simulink library "simlib_vpc_basic"  (R2022a)
settings: Solver=VariableStepAuto  StartTime=0.0  StopTime=10.0  RelTol=1e-3
undefined symbols (not defined in the file or in its folder): __PRM__SERIALIZED__DATA__, Ad, Camera, Pinhole, RBM, RRBM, VMO, VPC
libraries: $bdroot x10, simlib_vpc_coremath x5
(part 1 of 2)
settings Model: Creator=marco  LastModifiedBy=marco
settings SolverCC: AlgebraicLoopSolver=TrustRegion
settings DebuggingCC: UnconnectedInputMsg=warning  UnconnectedOutputMsg=warning  UnconnectedLineMsg=warning  SFMachineParentedDataDiag=warning
settings RTWCC: DLArmComputeVersion=19.05

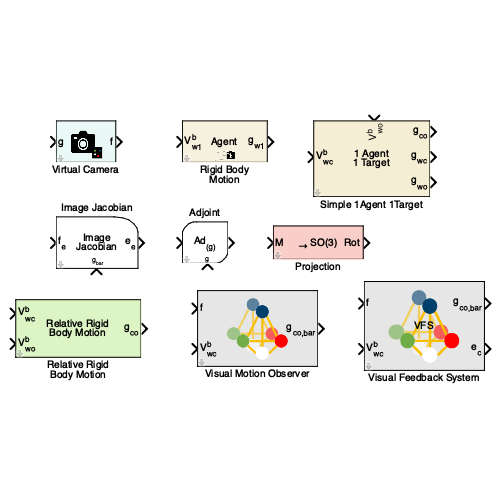
[thumbnail: Simulink's stored preview of the top-level diagram]
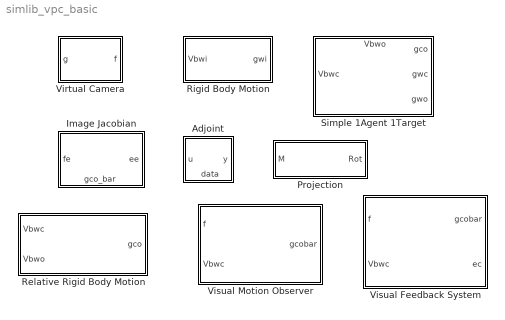
== system simlib_vpc_basic ==
  Adjoint : Subsystem  BlockKeywords=__PRM__SERIALIZED__DATA__:Ad  TreatAsAtomicUnit=on  mask(Adjoint Matrix [V1]){adjointtype=pose}
      mask prompts: adjointtype "Adjoint matrix is based on:"
      mask help:
      | Multiplies the Adjoint matrix with the input.
      | To calculate the Adjoint matrix, the position, orientation, or full pose must be given.
      settings: PortSchema="{\"entries\":[{\"content\":{\"sides\":[{\"content\":{\"connectorIds\":[\"In1\"]},\"type\":\"ConnectorPlacement.EquallySpacedRectSide\",\"uuid\":\"7e2da421-add1-40b5-9446-7b0ea0a4f10f\"},{\"content\":{\"connectorIds\":[\"Out1\"],\"side\":\"RIGHT\"},\"type\":\"ConnectorPlacement.EquallySpacedRectSide\",\"uuid\":\"b0158e1e-600a-48e8-a911-48a3898aac4e\"},{\"content\":{\"connectorIds\":[],\"side\":\"TOP\"},\"type\":\"ConnectorPlacement.EquallySpacedRectSide\",\"uuid\":\"4bc828d1-dee2-499b-9d21-a07f027570ae\"},{\"content\":{\"connectorIds\":[\"In2\"],\"side\":\"BOTTOM\"},\"type\":\"ConnectorPlacement.EquallySpacedRectSide\",\"uuid\":\"beed8369-7b41-42da-9d64-0cf6bc349210\"},{\"content\":{\"connectorIds\":[],\"side\":\"HIDDEN\"},\"type\":\"ConnectorPlacement.EquallySpacedRectSide\",\"uuid\":\"5ea700d9-1fcc-4187-8674-17f5733302d7\"}]},\"type\":\"ConnectorPlacement.EquallySpacedConnector\",\"uuid\":\"feef5c4e-af92-4970-8f4b-9fe20ba05ac5\"}],\"packageUris\":[\"http://schema.mathworks.com/mf0/Connector/R2020b\"],\"version\":\"1.0\"}"
      mask Help:
      | Refer to:
      | T. Hatanaka, N. Chopra, M. Fujita, and M. W. Spong, <i>Passivity-based Control and Estimation in Networked Robotics</i>, ser. Communications and Control Engineering. Springer, 2015.
      mask TypeOptions adjointtype: pose | position | orientation
      mask Display:
      | % Glitch in Matlab: If you define a line whose starting point and end point
      | % is equal, then the entire mask block is plotted in bold
      | plot([0,0],[0,0])
      | 
      | % Draw box
      | indent = 0.3;
      | ang=[0:0.2:pi/2, pi/2];
      | plot([0,1-indent],[0,0])
      | xp=indent*sin(ang)+1-indent;
      | yp=indent-indent*cos(ang);
      | plot(xp,yp);
      | plot([1,1,indent],[indent,1,1])
      | xp=indent-indent*sin(ang);
      | yp=1-indent+indent*cos(ang);
      | plot(xp,yp);
      | plot([0,0],[1-indent,0])
      | 
      | % Write label & ports
      | adjointtype = get_param(gcb, 'adjointtype');
      | porttype = '';
      | switch adjointtype
      |     case 'pose'
      |         disp('Ad_{(g)}','texmode','on')
      |         porttype = 'g';
      |     case 'position'
      |         disp('Ad_{(p)}','texmode','on')
      |         porttype = 'p';
      |     case 'orientation'
      |         disp('Ad_{(R)}','texmode','on')
      |         porttype = 'R';
      | end
      | switch get_param(gcb,'Orientation')
      |     case 'right'
      |         text(0.5,0.2,['\fontsize{7}' porttype],'texmode','on')
      |     case 'down'
      |         text(0.05,0.6,['\fontsize{7}' porttype],'texmode','on')
      |     case 'left'
      |         text(0.5,0.95,['\fontsize{7}' porttype],'texmode','on')
      |     case 'up'
      |         text(0.85,0.6,['\fontsize{7}' porttype],'texmode','on')
      | end
  Image Jacobian : Subsystem  TreatAsAtomicUnit=on  mask(Image Jacobian [V1]){po=[0, 10*sqrt(3), 0;15, -5*sqrt(3), 0;-15, -5*sqrt(3), 0;0, 0, 10*sqrt(6)]./100, lambda=0.0041}
      mask prompts: po "Feature point position coordinates (fixed in object frame Σo) [m]"; lambda "Focal length λ [m]"
      mask help:
      | Calculates the estimation error from the visual measurement error.
      | To that regard, the <i>Image Jacobian</i> is calculated, which itself depends on the VMO-estimate of the pose <i>gco</i>.
      |
      | Note: The focal length and feature point position coordinates in the object frame must be exactly known.
      settings: PortSchema="{\"entries\":[{\"content\":{\"sides\":[{\"content\":{\"connectorIds\":[\"In1\"]},\"type\":\"ConnectorPlacement.EquallySpacedRectSide\",\"uuid\":\"3d122c75-6063-48d0-bdc6-e48d95f4f0df\"},{\"content\":{\"connectorIds\":[\"Out1\"],\"side\":\"RIGHT\"},\"type\":\"ConnectorPlacement.EquallySpacedRectSide\",\"uuid\":\"6f2baba1-0bbd-4647-86ee-c97990dc6bd4\"},{\"content\":{\"connectorIds\":[],\"side\":\"TOP\"},\"type\":\"ConnectorPlacement.EquallySpacedRectSide\",\"uuid\":\"e6bc68d2-46ec-4597-a68e-7f59d26336ee\"},{\"content\":{\"connectorIds\":[\"In2\"],\"side\":\"BOTTOM\"},\"type\":\"ConnectorPlacement.EquallySpacedRectSide\",\"uuid\":\"b2d95be7-b34a-40bf-916a-28f2d4974c3e\"},{\"content\":{\"connectorIds\":[],\"side\":\"HIDDEN\"},\"type\":\"ConnectorPlacement.EquallySpacedRectSide\",\"uuid\":\"d66c6085-c61f-489e-b38a-36804ae2ee0b\"}]},\"type\":\"ConnectorPlacement.EquallySpacedConnector\",\"uuid\":\"9cb4cf54-89e1-4d8f-a4cb-7cce930f6af0\"}],\"packageUris\":[\"http://schema.mathworks.com/mf0/Connector/R2020b\"],\"version\":\"1.0\"}"
      mask Help:
      | Refer to:
      | T. Hatanaka, N. Chopra, M. Fujita, and M. W. Spong, <i>Passivity-based Control and Estimation in Networked Robotics</i>, ser. Communications and Control Engineering. Springer, 2015.
      mask Display:
      | % Glitch in Matlab: If you define a line whose starting point and end point
      | % is equal, then the entire mask block is plotted in bold
      | plot([0,0],[0,0])
      | 
      | % Draw box
      | indent = 0.3;
      | ang=[0:0.3:pi/2, pi/2];
      | xp=indent*cos(ang)+1-indent;
      | yp=indent*sin(ang)+1-indent;
      | plot([1,1,0,0,1-indent],[1-indent,0,0,1,1])
      | plot(xp,yp);
      | 
      | % Write label
      | % disp('J^{\spadesuit}(g_{co,bar})','texmode','on')
      | fprintf('Image\nJacobian','texmode','on')
      | 
      | % Label ports
      | port_label('input',1,'f_e','texmode','on')
      | % port_label('input',2,'g_{co,bar}','texmode','on')
      | text(0.45,0.2,'\fontsize{7}g_{bar}','texmode','on')
      | port_label('output',1,'e_e','texmode','on')
  Projection : Subsystem  TreatAsAtomicUnit=on  mask(Rotation Projection [V1]){projectiontype=averaging, inputtype=rotation matrix}
      mask prompts: projectiontype "Type of rotation projection:"; inputtype "Type of rotation input:"
      mask help:
      | This block projects an arbitrary matrix M [size 3x3] to the closest rotation matrix in SO3.
      |
      | Note:
      | Due to integration, a rotation matrix might only be "rotation"-like, as the determinant might change.
      | A real rotation matrix is orthogonal and has always determinant 1.
      | This block projects the input-matrix M to the closest rotation matrix R with such properties.
      mask Help:
      | Refer to:
      | T. Hatanaka, N. Chopra, M. Fujita, and M. W. Spong, <i>Passivity-based Control and Estimation in Networked Robotics</i>, ser. Communications and Control Engineering. Springer, 2015.
      mask TypeOptions projectiontype: averaging
      mask TypeOptions inputtype: rotation matrix | pose
      mask Display:
      | % Glitch in Matlab: If you define a line whose starting point and end point
      | % is equal, then the entire mask block is plotted in bold
      | plot([0,0],[0,0])
      | 
      | % Draw Box
      | plot([0,1,1,0,0],[0,0,1,1,0])
      | 
      | % Write label
      | disp('\rightarrow SO(3)','texmode','on')
      | 
      | % Label ports
      | inputtype = get_param(gcb, 'inputtype');
      | switch inputtype
      |     case 'rotation matrix'
      |         port_label('input',1,'M','texmode','on')
      |         port_label('output',1,'Rot','texmode','on')
      |     case 'pose'
      |         port_label('input',1,'g_M','texmode','on')
      |         port_label('output',1,'g','texmode','on')
      | end
  Relative Rigid Body Motion : Subsystem  BlockKeywords=__PRM__SERIALIZED__DATA__:RRBM  mask(Relative Rigid Body Motion Block [V1]){gco0=eye(4), projection=on, show_dgco=off}
      mask prompts: gco0 "Initial condition gco(0):"; projection "Use projection"; show_dgco "Show dgco"
      mask help: Relative rigid body motion of agent A as it can be observed from agent B.
      mask init:
      | block = find_system(gcb,'LookUnderMasks','on',...
      |     'FollowLinks','on','Name','Projection');
      | 
      | if projection && isempty(block) % Turn on projection
      |     % Delete lines
      |     delete_line(gcb,'Integrator/1','gco/1')
      |     delete_line(gcb,'Integrator/1','rrbm/3')
      |     
      |     % Add block
      |     add_block([bdroot(gcb),'/Projection'],[gcb,'/Projection'],'inputtype','pose');
      |     
      |     % Connect lines
      |     add_line(gcb,'Integrator/1','Projection/1','autorouting','smart')
      |     add_line(gcb,'Projection/1','gco/1','autorouting','smart')
      |     add_line(gcb,'Projection/1','rrbm/3','autorouting','smart')
      | elseif ~projection && ~isempty(block) % Turn off projection
      |     % Delete lines
      |     delete_line(gcb,'Integrator/1','Projection/1')
      |     delete_line(gcb,'Projection/1','gco/1')
      |     delete_line(gcb,'Projection/1','rrbm/3')
      | 
      |     % Delete block
      |     delete_block(block);
      | 
      |     % Connect blocks
      |     add_line(gcb,'Integrator/1','gco/1','autorouting','smart')
      |     add_line(gcb,'Integrator/1','rrbm/3','autorouting','smart')
      | end
      | 
      | % Show dgco output
      | if show_dgco
      |     % Add block & lines
      |     try; add_block('built-in/Outport',[gcb,'/dgco'],'Port','2','Position',[510 193 540 207]); end;
      |     try; add_line(gcb,'rrbm/1','dgco/1','autorouting','smart'); end;
      | else
      |     % Delete block & lines
      |     dgcoblock = find_system(gcb,'SearchDepth','1','LookUnderMasks','on',...
      |         'FollowLinks','on','Name','dgco');
      |     try; delete_line(gcb,'rrbm/1','dgco/1'); end;
      |     try; delete_block(dgcoblock); end;
      | end
      settings: MinAlgLoopOccurrences=on
      mask Help:
      | Refer to:
      | T. Hatanaka, N. Chopra, M. Fujita, and M. W. Spong, <i>Passivity-based Control and Estimation in Networked Robotics</i>, ser. Communications and Control Engineering. Springer, 2015.
      mask TypeOptions gco0: Integrator/InitialCondition
      mask DialogControl show_dgco Tooltip: If on, the internal state derivative of gco will be shown as an output
      mask Display:
      | % Glitch in Matlab: If you define a line whose starting point and end point
      | % is equal, then the entire mask block is plotted in bold
      | plot([0,0],[0,0])
      | 
      | % Draw Box
      | plot([0,1,1,0,0],[0,0,1,1,0])
      | 
      | % Write label
      | fprintf('Relative Rigid\nBody Motion','texmode','on')
      | 
      | % Label ports
      | port_label('input',1,'V^{b}_{wc}','texmode','on')
      | port_label('input',2,'V^{b}_{wo}','texmode','on')
      | port_label('output',1,'g_{co}','texmode','on')
      | if strcmp(get_param(gcb,'show_dgco'),'on')
      |     port_label('output',2,'dg_{co}','texmode','on')
      | end
  Rigid Body Motion : Subsystem  BlockKeywords=__PRM__SERIALIZED__DATA__:RBM  mask(Rigid Body Motion Block [V1]){rbmtype=agent, agentnumber=1, projection=on, show_dg=off, g0=eye(4)}
      mask prompts: rbmtype "Type:"; agentnumber "#"; projection "Use projection"; show_dg "Show derivative dg"; g0 "Initial condition g(0):"
      mask help:
      | Implements a simple (single-integrator-type) rigid body motion model.
      | The RBM type in the parameter pane is just for a better visualization purpose and does not have any effect on the dynamics, but the block mask appearance.
      mask init:
      | block = find_system(gcb,'LookUnderMasks','on',...
      |     'FollowLinks','on','Name','Projection');
      | 
      | if projection && isempty(block) % Turn on projection
      |     % Delete lines
      |     delete_line(gcb,'Integrator/1','gwi/1')
      |     delete_line(gcb,'Integrator/1','rbm/2')
      |     
      |     % Add block
      |     add_block([bdroot(gcb),'/Projection'],[gcb,'/Projection'],'inputtype','pose');
      |     
      |     % Connect lines
      |     add_line(gcb,'Integrator/1','Projection/1','autorouting','smart')
      |     add_line(gcb,'Projection/1','gwi/1','autorouting','smart')
      |     add_line(gcb,'Projection/1','rbm/2','autorouting','smart')
      | elseif ~projection && ~isempty(block) % Turn off projection
      |     % Delete lines
      |     delete_line(gcb,'Integrator/1','Projection/1')
      |     delete_line(gcb,'Projection/1','gwi/1')
      |     delete_line(gcb,'Projection/1','rbm/2')
      | 
      |     % Delete block
      |     delete_block(block);
      | 
      |     % Connect blocks
      |     add_line(gcb,'Integrator/1','gwi/1','autorouting','smart')
      |     add_line(gcb,'Integrator/1','rbm/2','autorouting','smart')
      | end
      | 
      | % Show derivative output dg
      | if show_dg
      |     % Add block & lines
      |     try; add_block('built-in/Outport',[gcb,'/dgwi'],'Port','2','Position',[515 203 545 217]); end;
      |     try; add_line(gcb,'rbm/1','dgwi/1','autorouting','smart'); end;
      | else
      |     % Delete block & lines
      |     dgwiblock = find_system(gcb,'SearchDepth','1','LookUnderMasks','on',...
      |         'FollowLinks','on','Name','dgwi');
      |     try; delete_line(gcb,'rbm/1','dgwi/1'); end;
      |     try; delete_block(dgwiblock); end;
      | end
      settings: MinAlgLoopOccurrences=on
      mask Help:
      | Refer to:
      | T. Hatanaka, N. Chopra, M. Fujita, and M. W. Spong, <i>Passivity-based Control and Estimation in Networked Robotics</i>, ser. Communications and Control Engineering. Springer, 2015.
      mask TypeOptions rbmtype: agent | target
      mask Callback rbmtype:
      | rbmtype = get_param(gcb,'rbmtype');
      | 
      | switch rbmtype
      |     case 'agent'
      |         % Turn on number field
      |         set_param(gcb,'MaskVisibilities',{'on';'on';'on';'on';'on'});
      |     case 'target'
      |         % Turn off number field
      |         set_param(gcb,'MaskVisibilities',{'on';'off';'on';'on';'on'});
      |         % Set number in the invisible field to 0
      |         % set_param(gcb,'agentnumber','0');
      | end
      mask Display:
      | % Glitch in Matlab: If you define a line whose starting point and end point
      | % is equal, then the entire mask block is plotted in bold
      | plot([0,0],[0,0])
      | 
      | % Draw Box
      | plot([0,1,1,0,0],[0,0,1,1,0])
      | 
      | % Write label
      | rbmtype = get_param(gcb, 'rbmtype');
      | switch rbmtype
      |     case 'agent'
      |         agentnumber = get_param(gcb, 'agentnumber');
      |         disp('Agent','texmode','on')
      | 
      |         % Image
      |         p=get_param(gcb,'Position');
      |         size = min(p(3:4)-p(1:2));
      |         blkscale = abs((p(3)-p(1)) / (p(4)-p(2)));
      |         if abs((p(3)-p(1))) > abs((p(4)-p(2))) % block is horizontal
      |             scale = .5*[1/blkscale .6];
      |         else % block is vertical
      |             scale = .5*[1 .6*blkscale];
      |         end
      |         pos = [1-scale(1) 0.1]/2;
      |         image('ico_agent.png',[pos scale],'off')
      |     case 'target'
      |         agentnumber = 0;
      |         disp('Target','texmode','on')
      | 
      |         % Image
      |         p=get_param(gcb,'Position');
      |         size = min(p(3:4)-p(1:2));
      |         blkscale = abs((p(3)-p(1)) / (p(4)-p(2)));
      |         if abs((p(3)-p(1))) > abs((p(4)-p(2))) % block is horizontal
      |             scale = .5*[1/blkscale .6];
      |         else % block is vertical
      |             scale = .5*[1 .6*blkscale];
      |         end
      |         pos = [1-scale(1) 0.1]/2;
      |         image('ico_target.png',[pos scale],'off')
      | end
      | 
      | % Label ports
      | port_label('input',1,['V^{b}_{w' num2str(agentnumber) '}'],'texmode','on')
      | port_label('output',1,['g_{w' num2str(agentnumber) '}'],'texmode','on')
      | if strcmp(get_param(gcb, 'show_dg'),'on')
      |     port_label('output',2,['dg_{w' num2str(agentnumber) '}'],'texmode','on')
      | end
  Simple 1Agent 1Target : Subsystem  mask(Simple 1Agent 1 Target block [V1]){gwc0=eye(4), projectionAgent=on, gwo0=eye(4), projectionTarget=on, showgwc=on, showdgwc=off, showgwo=on, showdgwo=off}
      mask prompts: gwc0 "Initial condition gwc(0):"; projectionAgent "Use projection"; gwo0 "Initial condition gwo(0):"; projectionTarget "Use projection"; showgwc "Output gwc"; showdgwc "Output dgwc"; showgwo "Output gwo"; showdgwo "Output dgwo"
      mask help: Implements a simple relative rigid body motion block with one target and one agent.
      mask init:
      | % Blocks
      | gwcblock = find_system(gcb,'LookUnderMasks','on',...
      |     'FollowLinks','on','Name','gwc');
      | dgwcblock = find_system(gcb,'LookUnderMasks','on',...
      |     'FollowLinks','on','Name','dgwc');
      | gwoblock = find_system(gcb,'LookUnderMasks','on',...
      |     'FollowLinks','on','Name','gwo');
      | dgwoblock = find_system(gcb,'LookUnderMasks','on',...
      |     'FollowLinks','on','Name','dgwo');
      | 
      | portnum = 2;
      | 
      | if showgwc % Output gwc
      |     % Add block
      |     try; add_block('built-in/Outport',[gcb,'/gwc'],'Position',[380 128 410 142],'Port',num2str(portnum)); end;
      |     portnum = portnum + 1;
      |     % Connect lines
      |     try; add_line(gcb,'Agent/1','gwc/1','autorouting','smart'); end;
      | else % Hide gwc
      |     % Delete lines
      |     try; delete_line(gcb,'Agent/1','gwc/1'); end;
      |     % Delete block
      |     try; delete_block(gwcblock); end;
      | end
      | 
      | if showdgwc % Output dgwc
      |     % Pass argument to agent block
      |     set_param([gcb,'/Agent'],'show_dg','on')
      |     % Add block
      |     try; add_block('built-in/Outport',[gcb,'/dgwc'],'Position',[200 148 230 162],'Port',num2str(portnum)); end;
      |     portnum = portnum + 1;
      |     % Connect lines
      |     try; add_line(gcb,'Agent/2','dgwc/1','autorouting','smart'); end;
      | else % Hide dgwc
      |     % Delete lines
      |     try; delete_line(gcb,'Agent/2','dgwc/1'); end;
      |     % Delete block
      |     try; delete_block(dgwcblock); end;
      |     % Pass argument to agent block
      |     set_param([gcb,'/Agent'],'show_dg','off')
      | end
      | 
      | if showgwo % Output gwc
      |     % Add block
      |     try; add_block('built-in/Outport',[gcb,'/gwo'],'Position',[380 48 410 62],'Port',num2str(portnum)); end;
      |     portnum = portnum + 1;
      |     % Connect lines
      |     try; add_line(gcb,'Target/1','gwo/1','autorouting','smart'); end;
      | else % Hide gwc
      |     % Delete lines
      |     try; delete_line(gcb,'Target/1','gwo/1'); end;
      |     % Delete block
      |     try; delete_block(gwoblock); end;
      | end
      | 
      | if showdgwo % Output dgwo
      |     % Pass argument to target block
      |     set_param([gcb,'/Target'],'show_dg','on')
      |     % Add block
      |     try; add_block('built-in/Outport',[gcb,'/dgwo'],'Position',[200 63 230 77],'Port',num2str(portnum)); end;
      |     portnum = portnum + 1;
      |     % Connect lines
      |     try; add_line(gcb,'Target/2','dgwo/1','autorouting','smart'); end;
      | else % Hide dgwo
      |     % Delete lines
      |     try; delete_line(gcb,'Target/2','dgwo/1'); end;
      |     % Delete block
      |     try; delete_block(dgwoblock); end;
      |     % Pass argument to agent block
      |     set_param([gcb,'/Target'],'show_dg','off')
      | end
      settings: PortSchema="{\"entries\":[{\"content\":{\"sides\":[{\"content\":{\"connectorIds\":[\"In1\"]},\"type\":\"ConnectorPlacement.EquallySpacedRectSide\",\"uuid\":\"51848c78-49bf-4d69-8138-12848c04a52b\"},{\"content\":{\"connectorIds\":[\"Out1\",\"Out2\",\"Out3\"],\"side\":\"RIGHT\"},\"type\":\"ConnectorPlacement.EquallySpacedRectSide\",\"uuid\":\"a2771237-d1b3-407b-8d53-6a34779e1c0e\"},{\"content\":{\"connectorIds\":[\"In2\"],\"side\":\"TOP\"},\"type\":\"ConnectorPlacement.EquallySpacedRectSide\",\"uuid\":\"c6712b15-7cf3-4a58-80e7-6bd7851abb53\"},{\"content\":{\"connectorIds\":[],\"side\":\"HIDDEN\"},\"type\":\"ConnectorPlacement.EquallySpacedRectSide\",\"uuid\":\"8616ed9a-8306-41f0-bffd-55839930ff42\"}]},\"type\":\"ConnectorPlacement.EquallySpacedConnector\",\"uuid\":\"4f48229c-43f3-4c05-9119-4c52932f0077\"}],\"packageUris\":[\"http://schema.mathworks.com/mf0/Connector/R2020b\"],\"version\":\"1.0\"}"
      mask Help:
      | Refer to:
      | T. Hatanaka, N. Chopra, M. Fujita, and M. W. Spong, <i>Passivity-based Control and Estimation in Networked Robotics</i>, ser. Communications and Control Engineering. Springer, 2015.
      mask TypeOptions gwc0: Agent/g0
      mask TypeOptions projectionAgent: Agent/projection
      mask TypeOptions gwo0: Target/g0
      mask TypeOptions projectionTarget: Target/projection
      mask DialogControl AgentParameters Prompt: Agent Parameters
      mask DialogControl TargetParameters Prompt: Target Parameters
      mask DialogControl OutputPorts Prompt: Auxiliary outputs
      mask Display:
      | % Glitch in Matlab: If you define a line whose starting point and end point
      | % is equal, then the entire mask block is plotted in bold
      | plot([0,0],[0,0])
      | 
      | % Draw Box
      | plot([0,1,1,0,0],[0,0,1,1,0])
      | 
      | % Write label
      | fprintf('1 Agent\n1 Target','texmode','on')
      | 
      | % Label ports
      | port_label('input',1,'V^{b}_{wc}','texmode','on')
      | port_label('input',2,'V^{b}_{wo}','texmode','on')
      | port_label('output',1,'g_{co}','texmode','on')
      | 
      | % Label dynamic output ports
      | portnumber = 2;
      | if strcmp(get_param(gcb, 'showgwc'),'on')
      |     port_label('output',portnumber,'g_{wc}','texmode','on')
      |     portnumber = portnumber + 1;
      | end
      | if strcmp(get_param(gcb, 'showdgwc'),'on')
      |     port_label('output',portnumber,'dg_{wc}','texmode','on')
      |     portnumber = portnumber + 1;
      | end
      | if strcmp(get_param(gcb, 'showgwo'),'on')
      |     port_label('output',portnumber,'g_{wo}','texmode','on')
      |     portnumber = portnumber + 1;
      | end
      | if strcmp(get_param(gcb, 'showdgwo'),'on')
      |     port_label('output',portnumber,'dg_{wo}','texmode','on')
      |     portnumber = portnumber + 1;
      | end
  Virtual Camera : Subsystem  BlockKeywords=__PRM__SERIALIZED__DATA__:Camera  TreatAsAtomicUnit=on  mask(Virtual Camera model [V1]){camtype=Pinhole, po=[0, 10*sqrt(3), 0;15, -5*sqrt(3), 0;-15, -5*sqrt(3), 0;0, 0, 10*sqrt(6)]./100, lambda=0.0041}
      mask prompts: camtype "Camera type"; po "Feature point position coordinates (fixed in object frame Σo) [m]"; lambda "Focal length λ [m]"
      mask help:
      | A simple virtual camera model.
      | Outputs feature points in image-coordinates.
      |
      | Note: So far, only a virtual "Pinhole" camera model is implemented.
      mask Help:
      | Refer to:
      | T. Hatanaka, N. Chopra, M. Fujita, and M. W. Spong, <i>Passivity-based Control and Estimation in Networked Robotics</i>, ser. Communications and Control Engineering. Springer, 2015.
      mask TypeOptions camtype: Pinhole
      mask Display:
      | % Glitch in Matlab: If you define a line whose starting point and end point
      | % is equal, then the entire mask block is plotted in bold
      | plot([0,0],[0,0])
      | 
      | % Draw Box
      | plot([0,1,1,0,0],[0,0,1,1,0])
      | 
      | % Write label
      | % disp('Camera','texmode','on')
      | p=get_param(gcb,'Position');
      | size = min(p(3:4)-p(1:2));
      | blkscale = abs((p(3)-p(1)) / (p(4)-p(2)));
      | if abs((p(3)-p(1))) > abs((p(4)-p(2))) % block is horizontal
      |     scale = .8*[1/blkscale 1];
      | else % block is vertical
      |     scale = .8*[1 blkscale];
      | end
      | pos = [1-scale(1) 1-scale(2)]./2;
      | image('ico_vis.png',[pos scale],'off')
      | 
      | % Label ports
      | port_label('input',1,'g','texmode','on')
      | port_label('output',1,'f','texmode','on')
  Visual Feedback System : Subsystem  BlockKeywords=__PRM__SERIALIZED__DATA__:VPC  mask(Visual Pursuit Control [V1]){gd_source=internal, gd_value=[eye(4,3),ones(4,1)], gcobar0=[eye(4,3), ones(4,1)], Ke_source=internal, Ke=5*eye(6), projection=on, camtype=Pinhole, fo=[0, 10*sqrt(3), 0;15, -5*sqrt(3), 0;-15, -5*sqrt(3), 0;0, 0, 10*sqrt(6)]./100, lambda=0.0041, show_Vbwo=off, show_ec=on, show_gce=off, show_ee=off, show_gee=off, show_e=off, show_nu=off, show_dgcobar=off, show_ue_aux=off}
      mask prompts: gd_source "Desired pose source:"; gd_value "Desired pose"; gcobar0 "Initial estimate gco_bar(0):"; Ke_source "Observer gain source:"; Ke "Observer gain Ke"; projection "Use projection"; camtype "Camera type"; fo "Feature point position coordinates (fixed in object frame Σo) [m]"; lambda "Camera focal length λ [m]"; show_Vbwo "estimated target velocity Vbwo"; show_ec "control error ec"; show_gce "control error gce"; show_ee "estimation error ee"; show_gee "estimation error gee"; show_e "total error e"; show_nu "nu"; show_dgcobar "estimation derivative"; show_ue_aux "feed-forward ue"
      mask help:
      | Visual Feedback System block.
      | Implements the visual pursuit control scheme. Has the visual motion observer block included.
      | Check parameters carefully.
      mask init:
      | % Switch gd: external <-> internal
      | port_number = 3;
      | switch gd_source
      |     case 1 % Make internal
      |         % Delete block & lines
      |         gd = find_system(gcb,'SearchDepth','1','LookUnderMasks','on',...
      |             'FollowLinks','on','Name','gd_inport');
      |         try; delete_line(gcb,'gd_inport/1','Relative Pose/1'); end;
      |         try; delete_block(gd); end;
      | 
      |         % Add block & lines
      |         try; add_block('built-in/Constant',[gcb,'/Desired Pose'],'Value','gd_value','Position',[190 -291 285 -269]); end;
      |         try; add_line(gcb,'Desired Pose/1','Relative Pose/1','autorouting','smart'); end;
      |     case 2 % Make external
      |         % Delete block & lines
      |         gd = find_system(gcb,'SearchDepth','1','LookUnderMasks','on',...
      |             'FollowLinks','on','Name','Desired Pose');
      |         try; delete_line(gcb,'Desired Pose/1','Relative Pose/1'); end;
      |         try; delete_block(gd); end;
      | 
      |         % Add block & lines
      |         try; add_block('built-in/Inport',[gcb,'/gd_inport'],'Port',num2str(port_number),'Position',[220 -287 250 -273]); end;
      |         port_number = port_number + 1;
      |         try; add_line(gcb,'gd_inport/1','Relative Pose/1','autorouting','smart'); end;
      | end
      | 
      | % Switch Ke: external <-> internal
      | switch Ke_source
      |     case 1 % Make internal
      |         % Delete block & lines
      |         Ke_inport = find_system(gcb,'SearchDepth','1','LookUnderMasks','on',...
      |             'FollowLinks','on','Name','Ke_inport');
      |         Ke_mult = find_system(gcb,'SearchDepth','1','LookUnderMasks','on',...
      |             'FollowLinks','on','Name','Ke_mult');
      |         try; delete_line(gcb,'Demux/2','Ke_mult/2'); end;
      |         try; delete_line(gcb,'Ke_inport/1','Ke_mult/1'); end;
      |         try; delete_line(gcb,'Ke_mult/1','Gain/1'); end;
      |         try; delete_block(Ke_mult); end;
      |         try; delete_block(Ke_inport); end;
      | 
      |         % Add block & lines
      |         try; add_block('built-in/Gain',[gcb,'/Ke_gain'],'Gain','Ke','Multiplication','Matrix(K*u) (u vector)','Position',[175 -48 250 28],'Orientation','left'); end;
      |         try; add_line(gcb,'Demux/2','Ke_gain/1','autorouting','smart'); end;
      |         try; add_line(gcb,'Ke_gain/1','Gain/1','autorouting','smart'); end;
      |     case 2 % Make external
      |         % Delete block & lines
      |         Ke_gain = find_system(gcb,'SearchDepth','1','LookUnderMasks','on',...
      |             'FollowLinks','on','Name','Ke_gain');
      |         try; delete_line(gcb,'Demux/2','Ke_gain/1'); end;
      |         try; delete_line(gcb,'Ke_gain/1','Gain/1'); end;
      |         try; delete_block(Ke_gain); end;
      | 
      |         % Add block & lines
      |         try; add_block('built-in/Inport',[gcb,'/Ke_inport'],'Position',[255 -42 285 -28],'Port',num2str(port_number),'Orientation','left'); end;
      |         port_number = port_number + 1;
      |         try; add_block('built-in/Product',[gcb,'/Ke_mult'],'Multiplication','Matrix(*)','Position',[160 -50 210 5],'Orientation','left'); end;
      |         try; add_line(gcb,'Ke_inport/1','Ke_mult/1','autorouting','smart'); end;
      |         try; add_line(gcb,'Demux/2','Ke_mult/2','autorouting','smart'); end;
      |         try; add_line(gcb,'Ke_mult/1','Gain/1','autorouting','smart'); end;
      | end
      | 
      | % Show / Hide: ue_aux
      | if show_ue_aux % Show input
      |     % Delete block & lines
      |     try; delete_line(gcb,'Gain/1','Gain_ue/1'); end;
      | 
      |     % Add block & lines
      |     try; add_block('built-in/Inport',[gcb,'/ue_aux'],'Port',num2str(port_number),'Position',[-150 -132 -120 -118]); end;
      |     try; add_block('built-in/sum',[gcb,'/sum_ue'],'IconShape','round','Position',[-90 -135 -70 -115],'Inputs','|++'); end;
      |     try; add_line(gcb,'ue_aux/1','sum_ue/1','autorouting','smart'); end;
      |     try; add_line(gcb,'Gain/1','sum_ue/2','autorouting','smart'); end;
      |     try; add_line(gcb,'sum_ue/1','Gain_ue/1','autorouting','smart'); end;
      | else % Hide input
      |     % Delete block & lines
      |     ue = find_system(gcb,'SearchDepth','1','LookUnderMasks','on',...
      |         'FollowLinks','on','Name','ue_aux');
      |     sumblock = find_system(gcb,'SearchDepth','1','LookUnderMasks','on',...
      |         'FollowLinks','on','Name','sum_ue');
      |     try; delete_line(gcb,'ue_aux/1','sum_ue/1'); end;
      |     try; delete_line(gcb,'Gain/1','sum_ue/2'); end;
      |     try; delete_line(gcb,'sum_ue/1','Gain_ue/1'); end;
      |     try; delete_block(ue); end;
      |     try; delete_block(sumblock); end;
      | 
      |     % Add block & lines
      |     try; add_line(gcb,'Gain/1','Gain_ue/1','autorouting','smart'); end;
      | end
      | 
      | 
      | %%%%%%%%%%%%%%%%%%
      | %% Outputs
      | %%%%%%%%%%%%%%%%%%
      | port_number = 2;
      | 
      | % Show / Hide: Vbwo
      | if show_Vbwo % Show output
      |     try add_block('built-in/Outport',[gcb,'/Vbwo,bar'],'Port',num2str(port_number),'Position',[35 -77 65 -63]); catch; end
      |     try add_line(gcb,'Gain_ue/1','Vbwo,bar/1','autorouting','smart'); catch; end
      |     port_number = port_number+1;
      | else % Hide output
      |     block = find_system(gcb,'SearchDepth','1','LookUnderMasks','on',...
      |         'FollowLinks','on','Name','Vbwo,bar');
      |     try delete_line(gcb,'Gain_ue/1','Vbwo,bar/1'); catch; end
      |     try delete_block(block); catch; end
      | end
      | 
      | % Show / Hide: ec
      | if show_ec % Show output
      |     % Add block & lines
      |     try add_block('built-in/Outport',[gcb,'/ec'],'Port',num2str(port_number),'Position',[515 -262 545 -248]); catch; end
      |     try add_line(gcb,'vec/1','ec/1','autorouting','smart'); catch; end
      |     port_number = port_number + 1;
      | else % Hide output
      |     % Delete block & lines
      |     block = find_system(gcb,'SearchDepth','1','LookUnderMasks','on',...
      |         'FollowLinks','on','Name','ec');
      |     try delete_line(gcb,'vec/1','ec/1'); catch; end
      |     try delete_block(block); catch; end
      | end
      | 
      | % Show / Hide: ee
      | if show_ee % Show output
      |     try; add_block('built-in/Outport',[gcb,'/ee'],'Port',num2str(port_number),'Position',[515 -122 545 -108]); end;
      |     port_number = port_number + 1;
      |     try; add_line(gcb,'Image Jacobian/1','ee/1','autorouting','smart'); end;
      | else % Hide output
      |     ee = find_system(gcb,'SearchDepth','1','LookUnderMasks','on',...
      |         'FollowLinks','on','Name','ee');
      |     try; delete_line(gcb,'Image Jacobian/1','ee/1'); end;
      |     try; delete_block(ee); end;
      | end
      | 
      | % Show / Hide: gce
      | if show_gce % Show output
      |     try; add_block('built-in/Outport',[gcb,'/gce'],'Port',num2str(port_number),'Position',[515 -332 545 -318]); end;
      |     port_number = port_number + 1;
      |     try; add_line(gcb,'Relative Pose/1','gce/1','autorouting','smart'); end;
      | else % Hide output
      |     gce = find_system(gcb,'SearchDepth','1','LookUnderMasks','on',...
      |         'FollowLinks','on','Name','gce');
      |     try; delete_line(gcb,'Relative Pose/1','gce/1'); end;
      |     try; delete_block(gce); end;
      | end
      | 
      | % Show / Hide: gee
      | if show_gee % Show output
      |     block = find_system(gcb,'SearchDepth','1','LookUnderMasks','on',...
      |         'FollowLinks','on','Name','Terminator_gee');
      |     try delete_line(gcb,'unvec/1','Terminator_gee/1'); catch; end
      |     try delete_block(block); catch; end
      |     try add_block('built-in/Outport',[gcb,'/gee'],'Port',num2str(port_number),'Position',[645 -62 675 -48]); catch; end
      |     try add_line(gcb,'unvec/1','gee/1','autorouting','smart'); catch; end
      |     port_number = port_number+1;
      | else % Hide output
      |     block = find_system(gcb,'SearchDepth','1','LookUnderMasks','on',...
      |         'FollowLinks','on','Name','gee');
      |     try delete_line(gcb,'unvec/1','gee/1'); catch; end
      |     try delete_block(block); catch; end
      |     try add_block('built-in/Terminator',[gcb,'/Terminator_gee'],'Position',[645 -62 675 -48]); catch; end
      |     try add_line(gcb,'unvec/1','Terminator_gee/1','autorouting','smart'); catch; end
      | end
      | 
      | % Show / Hide: e
      | if show_e % Show output
      |     try; add_block('built-in/Outport',[gcb,'/e'],'Port',num2str(port_number),'Position',[660 -177 690 -163]); end;
      |     port_number = port_number + 1;
      |     try; add_line(gcb,'Vector Concatenate/1','e/1','autorouting','smart'); end;
      | else % Hide output
      |     e = find_system(gcb,'SearchDepth','1','LookUnderMasks','on',...
      |         'FollowLinks','on','Name','e');
      |     try; delete_line(gcb,'Vector Concatenate/1','e/1'); end;
      |     try; delete_block(e); end;
      | end
      | 
      | % Show / Hide: nu
      | if show_nu % Show output
      |     try; add_block('built-in/Outport',[gcb,'/nu'],'Port',num2str(port_number),'Position',[860 -242 890 -228]); end;
      |     port_number = port_number + 1;
      |     try; add_line(gcb,'Matrix Multiply/1','nu/1','autorouting','smart'); end;
      | else % Hide output
      |     nu = find_system(gcb,'SearchDepth','1','LookUnderMasks','on',...
      |         'FollowLinks','on','Name','nu');
      |     try; delete_line(gcb,'Matrix Multiply/1','nu/1'); end;
      |     try; delete_block(nu); end;
      | end
      | 
      | % Show / Hide: dgcobar
      | if show_dgcobar % Show output
      |     % Pass argument to rrbm block
      |     set_param([gcb,'/RRBM'],'show_dgco','on')
      |     % Add block & lines
      |     try; add_block('built-in/Outport',[gcb,'/dgcobar'],'Port',num2str(port_number),'Position',[225 -77 255 -63]); end;
      |     try; add_line(gcb,'RRBM/2','dgcobar/1','autorouting','smart'); end;
      | else
      |     % Delete block & lines
      |     dgcobarblock = find_system(gcb,'SearchDepth','1','LookUnderMasks','on',...
      |         'FollowLinks','on','Name','dgcobar');
      |     try; delete_line(gcb,'RRBM/2','dgcobar/1'); end;
      |     try; delete_block(dgcobarblock); end;
      |     % Pass argument to rrbm block
      |     set_param([gcb,'/RRBM'],'show_dgco','off')
      | end
      settings: MinAlgLoopOccurrences=on
      mask Help:
      | Refer to:
      | T. Hatanaka, N. Chopra, M. Fujita, and M. W. Spong, <i>Passivity-based Control and Estimation in Networked Robotics</i>, ser. Communications and Control Engineering. Springer, 2015.
      mask TypeOptions gd_source: internal | external
      mask Callback gd_source:
      | gd_source = get_param(gcb,'gd_source');
      | 
      | idx = find(strcmp(get_param(gcb,'MaskNames'),'gd_value'));
      | maskvis = get_param(gcb,'MaskVisibilities');
      | switch gd_source
      |     case 'internal' % Show gd field
      |         maskvis{idx} = 'on';
      |     case 'external' % Hide gd field
      |         maskvis{idx} = 'off';
      | end
      | set_param(gcb,'MaskVisibilities',maskvis);
      mask TypeOptions gcobar0: RRBM/gco0
      mask TypeOptions Ke_source: internal | external
      mask Callback Ke_source:
      | Ke_source = get_param(gcb,'Ke_source');
      | 
      | idx = find(strcmp(get_param(gcb,'MaskNames'),'Ke'));
      | maskvis = get_param(gcb,'MaskVisibilities');
      | switch Ke_source
      |     case 'internal' % Show Ke field
      |         maskvis{idx} = 'on';
      |     case 'external' % Hide Ke field
      |         maskvis{idx} = 'off';
      | end
      | set_param(gcb,'MaskVisibilities',maskvis);
      mask TypeOptions projection: RRBM/projection
      mask TypeOptions camtype: Virtual Camera/camtype
      mask TypeOptions fo: Virtual Camera/po
      mask TypeOptions lambda: Virtual Camera/lambda
      mask DialogControl VPCParameters Prompt: VPC Parameters
      mask DialogControl VMOParameters Prompt: VMO Parameters
      mask DialogControl CameraParameters Prompt: Camera Parameters
      mask DialogControl IOGroupVar Prompt: Show I/O
      mask DialogControl io_text Prompt: Tick the following checkboxes to show the corresponding inputs and outputs on the block.
      mask DialogControl Container7 Prompt: Outputs
      mask DialogControl show_gce Tooltip: If on, the pose control error gce will be shown at the output.
      mask DialogControl show_dgcobar Tooltip: If on, the estimation derivative dgcobar will be shown on the output.
      mask DialogControl Container8 Prompt: Inputs
      mask Display:
      | % Glitch in Matlab: If you define a line whose starting point and end point
      | % is equal, then the entire mask block is plotted in bold
      | plot([0,0],[0,0])
      | 
      | % Draw Box
      | plot([0,1,1,0,0],[0,0,1,1,0])
      | 
      | % Write label
      | p=get_param(gcb,'Position');
      | size = min(p(3:4)-p(1:2));
      | blkscale = abs((p(3)-p(1)) / (p(4)-p(2)));
      | if abs((p(3)-p(1))) > abs((p(4)-p(2))) % block is horizontal
      |     scale = .8*[1/blkscale 1];
      | else % block is vertical
      |     scale = .8*[1 blkscale];
      | end
      | pos = [1-scale(1) 1-scale(2)]./2;
      | image('ico_vmo.png',[pos scale],'off')
      | disp('VFS','texmode','on')
      | 
      | % Label input ports
      | port_label('input',1,'f','texmode','on')
      | port_label('input',2,'V^{b}_{wc}','texmode','on')
      | inport = 3;
      | if strcmp(get_param(gcb, 'gd_source'),'external')
      |     port_label('input',inport,'g_d','texmode','on')
      |     inport = inport + 1;
      | end
      | if strcmp(get_param(gcb, 'Ke_source'),'external')
      |     port_label('input',outport,'K_e','texmode','on')
      |     inport = inport + 1;
      | end
      | if strcmp(get_param(gcb, 'show_ue_aux'),'on')
      |     port_label('input',inport,'u_{e,aux}','texmode','on')
      |     inport = inport + 1;
      | end
      | 
      | % Label output ports
      | port_label('output',1,'g_{co,bar}','texmode','on')
      | outport = 2;
      | if strcmp(get_param(gcb, 'show_Vbwo'),'on')
      |     port_label('output',outport,'V^b_{wo,bar}','texmode','on')
      |     outport = outport+1;
      | end
      | if strcmp(get_param(gcb, 'show_ec'),'on')
      |     port_label('output',outport,'e_{c}','texmode','on')
      |     outport = outport+1;
      | end
      | if strcmp(get_param(gcb, 'show_ee'),'on')
      |     port_label('output',outport,'e_{e}','texmode','on')
      |     outport = outport+1;
      | end
      | if strcmp(get_param(gcb, 'show_gce'),'on')
      |     port_label('output',outport,'g_{ce}','texmode','on')
      |     outport = outport+1;
      | end
      | if strcmp(get_param(gcb, 'show_gee'),'on')
      |     port_label('output',outport,'g_{ee}','texmode','on')
      |     outport = outport+1;
      | end
      | if strcmp(get_param(gcb, 'show_e'),'on')
      |     port_label('output',outport,'e','texmode','on')
      |     outport = outport+1;
      | end
      | if strcmp(get_param(gcb, 'show_nu'),'on')
      |     port_label('output',outport,'\nu','texmode','on')
      |     outport = outport+1;
      | end
      | if strcmp(get_param(gcb, 'show_dgcobar'),'on')
      |     port_label('output',outport,'dg_{co,bar}','texmode','on')
      |     outport = outport+1;
      | end
  Visual Motion Observer : Subsystem  BlockKeywords=__PRM__SERIALIZED__DATA__:VMO  mask(Visual Motion Observer [V1]){show_ee=off, show_gee=off, show_Vbwo=off, show_dgcobar=off, show_ue_aux=off, gcobar0=[eye(4,3), ones(4,1)], projection=on, Ke_source=internal, Ke=5*eye(6), camtype=Pinhole, fo=[0, 10*sqrt(3), 0;15, -5*sqrt(3), 0;-15, -5*sqrt(3), 0;0, 0, 10*sqrt(6)]./100, lambda=0.0041}
      mask prompts: show_ee "estimation error ee"; show_gee "estimation error gee"; show_Vbwo "estimated target velocity Vbwo"; show_dgcobar "estimation derivative"; show_ue_aux "feed-forward ue"; gcobar0 "Initial estimate gco_bar(0):"; projection "Use projection"; Ke_source "Observer gain source:"; Ke "Observer gain Ke"; camtype "Camera type"; fo "Feature point position coordinates (fixed in object frame Σo) [m]"; lambda "Camera focal length λ [m]"
      mask help:
      | Visual Motion Observer Block.
      | Check parameters carefully.
      mask init:
      | % Blocks
      | ueblock = find_system(gcb,'SearchDepth','1','LookUnderMasks','on',...
      |     'FollowLinks','on','Name','ue_aux');
      | 
      | if show_ue_aux && isempty(ueblock) % Show ue inport
      |     % Delete line
      |     delete_line(gcb,'Gain/1','Gain_ue/1')
      |     % Add block
      |     port_number = 3;
      |     if Ke_source == 1 % Internal
      |         port_number = 3;
      |     else % External
      |         port_number = 4;
      |     end
      |     add_block('built-in/Inport',[gcb,'/ue_aux'],'Position',[155 278 185 292],'Port',num2str(port_number));
      |     add_block('built-in/sum',[gcb,'/sum_ue'],'Position',[215 275 235 295],'Inputs','|++');
      |     % Connect lines
      |     add_line(gcb,'ue_aux/1','sum_ue/1','autorouting','smart');
      |     add_line(gcb,'sum_ue/1','Gain_ue/1','autorouting','smart');
      |     add_line(gcb,'Gain/1','sum_ue/2','autorouting','smart')
      | elseif ~show_ue_aux && ~isempty(ueblock) % Hide ue inport
      |     sum_ue = find_system(gcb,'SearchDepth','1','LookUnderMasks','on',...
      |         'FollowLinks','on','Name','sum_ue');
      |     % Delete lines
      |     delete_line(gcb,'ue_aux/1','sum_ue/1')
      |     delete_line(gcb,'sum_ue/1','Gain_ue/1')
      |     delete_line(gcb,'Gain/1','sum_ue/2')
      |     % Delete block
      |     delete_block(ueblock);
      |     delete_block(sum_ue);
      |     % Add line
      |     add_line(gcb,'Gain/1','Gain_ue/1','autorouting','smart')
      | end
      | 
      | out_port = 2;
      | 
      | % Show Vbwo output
      | if show_Vbwo
      |     % Add block & lines
      |     try add_block('built-in/Outport',[gcb,'/Vbwo,bar'],'Port',num2str(out_port),'Position',[325 328 355 342]); catch; end
      |     try add_line(gcb,'Gain_ue/1','Vbwo,bar/1','autorouting','smart'); catch; end
      |     out_port = out_port+1;
      | else
      |     % Delete block & lines
      |     block = find_system(gcb,'SearchDepth','1','LookUnderMasks','on',...
      |         'FollowLinks','on','Name','Vbwo,bar');
      |     try delete_line(gcb,'Gain_ue/1','Vbwo,bar/1'); catch; end
      |     try delete_block(block); catch; end
      | end
      | 
      | % Show ee output
      | if show_ee
      |     % Add block & lines
      |     try add_block('built-in/Outport',[gcb,'/ee'],'Port',num2str(out_port),'Position',[800 218 830 232]); catch; end
      |     try add_line(gcb,'Image Jacobian/1','ee/1','autorouting','smart'); catch; end
      |     out_port = out_port+1;
      | else
      |     % Delete block & lines
      |     eeblock = find_system(gcb,'SearchDepth','1','LookUnderMasks','on',...
      |         'FollowLinks','on','Name','ee');
      |     try delete_line(gcb,'Image Jacobian/1','ee/1'); catch; end
      |     try delete_block(eeblock); catch; end
      | end
      | 
      | % Show gee output
      | if show_gee
      |     block = find_system(gcb,'SearchDepth','1','LookUnderMasks','on',...
      |         'FollowLinks','on','Name','Terminator_gee');
      |     try delete_line(gcb,'unvec/1','Terminator_gee/1'); catch; end
      |     try delete_block(block); catch; end
      |     try add_block('built-in/Outport',[gcb,'/gee'],'Port',num2str(out_port),'Position',[885 258 915 272]); catch; end
      |     try add_line(gcb,'unvec/1','gee/1','autorouting','smart'); catch; end
      |     out_port = out_port+1;
      | else
      |     block = find_system(gcb,'SearchDepth','1','LookUnderMasks','on',...
      |         'FollowLinks','on','Name','gee');
      |     try delete_line(gcb,'unvec/1','gee/1'); catch; end
      |     try delete_block(block); catch; end
      |     try add_block('built-in/Terminator',[gcb,'/Terminator_gee'],'Position',[875 255 895 275]); catch; end
      |     try add_line(gcb,'unvec/1','Terminator_gee/1','autorouting','smart'); catch; end
      | end
      | 
      | % Show estimation derivative dgcobar output
      | if show_dgcobar
      |     % Pass argument to rrbm block
      |     set_param([gcb,'/rrbm'],'show_dgco','on')
      |     % Add block & lines
      |     try; add_block('built-in/Outport',[gcb,'/dgcobar'],'Port',num2str(out_port),'Position',[505 333 535 347]); end;
      |     try; add_line(gcb,'rrbm/2','dgcobar/1','autorouting','smart'); end;
      | else
      |     % Delete block & lines
      |     dgcobarblock = find_system(gcb,'SearchDepth','1','LookUnderMasks','on',...
      |         'FollowLinks','on','Name','dgcobar');
      |     try; delete_line(gcb,'rrbm/2','dgcobar/1'); end;
      |     try; delete_block(dgcobarblock); end;
      |     % Pass argument to rrbm block
      |     set_param([gcb,'/rrbm'],'show_dgco','off')
      | end
      | 
      | 
      | % Switch Ke: external <-> internal
      | switch Ke_source
      |     case 1 % Make internal
      |         % Delete block & lines
      |         Ke_inport = find_system(gcb,'SearchDepth','1','LookUnderMasks','on',...
      |             'FollowLinks','on','Name','Ke_inport');
      |         Ke_mult = find_system(gcb,'SearchDepth','1','LookUnderMasks','on',...
      |             'FollowLinks','on','Name','Ke_mult');
      |         try; delete_line(gcb,'Image Jacobian/1','Ke_mult/2'); end;
      |         try; delete_line(gcb,'Ke_inport/1','Ke_mult/1'); end;
      |         try; delete_line(gcb,'Ke_mult/1','Gain/1'); end;
      |         try; delete_block(Ke_mult); end;
      |         try; delete_block(Ke_inport); end;
      | 
      |         % Add block & lines
      |         try; add_block('built-in/Gain',[gcb,'/Ke_gain'],'Gain','Ke','Multiplication','Matrix(K*u) (u vector)','Position',[415 347 490 423],'Orientation','left'); end;
      |         try; add_line(gcb,'Image Jacobian/1','Ke_gain/1','autorouting','smart'); end;
      |         try; add_line(gcb,'Ke_gain/1','Gain/1','autorouting','smart'); end;
      |     case 2 % Make external
      |         % Delete block & lines
      |         Ke_gain = find_system(gcb,'SearchDepth','1','LookUnderMasks','on',...
      |             'FollowLinks','on','Name','Ke_gain');
      |         try; delete_line(gcb,'Image Jacobian/1','Ke_gain/1'); end;
      |         try; delete_line(gcb,'Ke_gain/1','Gain/1'); end;
      |         try; delete_block(Ke_gain); end;
      | 
      |         % Add block & lines
      |         try; add_block('built-in/Inport',[gcb,'/Ke_inport'],'Position',[490 363 520 377],'Port','3','Orientation','left'); end;
      |         try; add_block('built-in/Product',[gcb,'/Ke_mult'],'Multiplication','Matrix(*)','Position',[405 359 450 406],'Orientation','left'); end;
      |         try; add_line(gcb,'Ke_inport/1','Ke_mult/1','autorouting','smart'); end;
      |         try; add_line(gcb,'Image Jacobian/1','Ke_mult/2','autorouting','smart'); end;
      |         try; add_line(gcb,'Ke_mult/1','Gain/1','autorouting','smart'); end;
      | end
      settings: MinAlgLoopOccurrences=on
      mask Help:
      | Refer to:
      | T. Hatanaka, N. Chopra, M. Fujita, and M. W. Spong, <i>Passivity-based Control and Estimation in Networked Robotics</i>, ser. Communications and Control Engineering. Springer, 2015.
      mask TypeOptions gcobar0: rrbm/gco0
      mask TypeOptions projection: rrbm/projection
      mask TypeOptions Ke_source: internal | external
      mask Callback Ke_source:
      | Ke_source = get_param(gcb,'Ke_source');
      | 
      | idx = find(strcmp(get_param(gcb,'MaskNames'),'Ke'));
      | maskvis = get_param(gcb,'MaskVisibilities');
      | switch Ke_source
      |     case 'internal' % Show Ke field
      |         maskvis{idx} = 'on';
      |     case 'external' % Hide Ke field
      |         maskvis{idx} = 'off';
      | end
      | set_param(gcb,'MaskVisibilities',maskvis);
      mask TypeOptions camtype: Virtual Camera/camtype
      mask DialogControl VMOParameters Prompt: VMO Parameters
      mask DialogControl IOGroupVar Prompt: Show I/O
      mask DialogControl io_text Prompt: Tick the following checkboxes to show the corresponding inputs and outputs on the block.
      mask DialogControl OutputGroupVar Prompt: Outputs
      mask DialogControl show_dgcobar Tooltip: If on, the estimation derivative dgcobar will be shown on the output.
      mask DialogControl InputGroupVar Prompt: Inputs
      mask DialogControl show_ue_aux Tooltip: If on, the internal observer input is calculated as: ue = -Ke*ee + ue_aux. The last term represents the feed-forward input, which is necessary if e.g. a GP model is used.
      mask DialogControl CameraParameters Prompt: Camera Parameters
      mask Display:
      | % Glitch in Matlab: If you define a line whose starting point and end point
      | % is equal, then the entire mask block is plotted in bold
      | plot([0,0],[0,0])
      | 
      | % Draw Box
      | plot([0,1,1,0,0],[0,0,1,1,0])
      | 
      | % Write label
      | % disp('VMO','texmode','on')
      | p=get_param(gcb,'Position');
      | size = min(p(3:4)-p(1:2));
      | blkscale = abs((p(3)-p(1)) / (p(4)-p(2)));
      | if abs((p(3)-p(1))) > abs((p(4)-p(2))) % block is horizontal
      |     scale = .8*[1/blkscale 1];
      | else % block is vertical
      |     scale = .8*[1 blkscale];
      | end
      | pos = [1-scale(1) 1-scale(2)]./2;
      | image('ico_vmo.png',[pos scale],'off')
      | 
      | % Label input ports
      | port_label('input',1,'f','texmode','on')
      | port_label('input',2,'V^{b}_{wc}','texmode','on')
      | Ke_source = get_param(gcb, 'Ke_source');
      | port_number = 3;
      | switch Ke_source
      |     case 'internal'
      |     case 'external'
      |         port_label('input',3,'K_e','texmode','on')
      |         port_number = 4;
      | end
      | show_ue_aux = get_param(gcb, 'show_ue_aux');
      | if show_ue_aux == "on"
      |     port_label('input',port_number,'u_{e,aux}','texmode','on')
      | end
      | 
      | % Label output ports
      | port_label('output',1,'g_{co,bar}','texmode','on')
      | port_number = 2;
      | if strcmp(get_param(gcb, 'show_Vbwo'),'on')
      |     port_label('output',port_number,'V^b_{wo,bar}','texmode','on')
      |     port_number = port_number+1;
      | end
      | if strcmp(get_param(gcb, 'show_ee'),'on')
      |     port_label('output',port_number,'e_{e}','texmode','on')
      |     port_number = port_number+1;
      | end
      | if strcmp(get_param(gcb, 'show_gee'),'on')
      |     port_label('output',port_number,'g_{ee}','texmode','on')
      |     port_number = port_number+1;
      | end
      | if strcmp(get_param(gcb, 'show_dgcobar'),'on')
      |     port_label('output',port_number,'dg_{co,bar}','texmode','on')
      |     port_number = port_number+1;
      | end
